simulink model "minJerk"  (R2014b)
settings: Solver=FixedStepDiscrete  StartTime=0.0  StopTime=100  FixedStep=0.01  RelTol=1e-3
InitFcn:
  | Plant_IC=0.0;
  | Plant_Min=-100.0;
  | Plant_Max=100.0;
  | Compensator_Kp=10.0;
  | Compensator_Ki=1.0;
  | AutoCompensator_ThresHystMax=0.05;
  | AutoCompensator_ThresHystMin=0.005;
  | ErrorStatisticsTimeWindow=1.0;
undefined symbols (not defined in the file or in its folder): CompensatorState
libraries: simulink x1, powerlib_meascontrol x1, dspbuff3 x1, dspstat3 x1, discretizing x1
settings Model: Creator=Ugo Pattacini  LastModifiedBy=Ugo Pattacini
settings OptimizationCC: OptimizeModelRefInitCode=on  LifeSpan=1
settings RTWCC: SystemTargetFile=ert.tlc  GenCodeOnly=on  TemplateMakefile=ert_default_tmf  Description=Embedded Coder  GenerateReport=on  ProcessScript=ert_make_rtw_hook  BuildConfiguration=Faster Runs  IncludeHyperlinkInReport=on  LaunchReport=on  TargetLang=C++
settings CodeAppCC: IgnoreCustomStorageClasses=off
settings ERTTargetCC: TargetLangStandard=C++03 (ISO)  GenerateSampleERTMain=on  MultiInstanceERTCode=on  CodeInterfacePackaging=Reusable function  ERTCustomFileTemplate=example_file_process.tlc

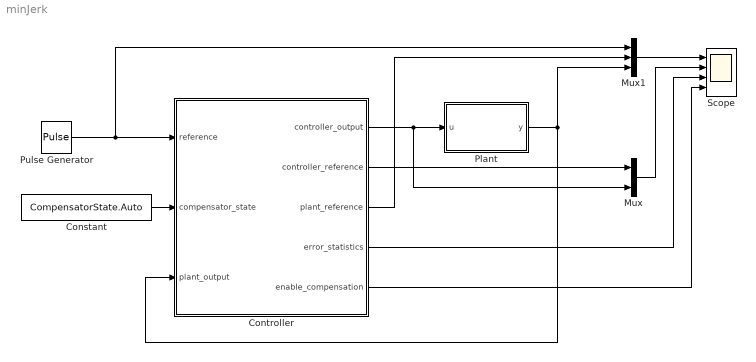
== system minJerk ==
  Constant : Constant  Value=CompensatorState.Auto  OutDataTypeStr=Enum: CompensatorState
  Controller : Subsystem
  Mux : Mux  Inputs=2
  Mux1 : Mux  Inputs=3
  Plant : Subsystem  TreatAsAtomicUnit=on  RTWFcnName=Plant
      settings: RTWFcnNameOpts=User specified
  Pulse Generator : DiscretePulseGenerator  PulseType=Time based  Period=20  PulseWidth=50
  Scope : Scope  NumInputPorts=4
      settings: TimeRange=100  YMin=-0.5~-2~0~-1  YMax=1.5~2~0.15~2
  wires:
  Pulse Generator/1 -> Mux1/1, Controller/1(reference)
  Controller/2(controller_reference) -> Mux/1
  Controller/3(plant_reference) -> Mux1/2
  Mux1/1 -> Scope/1
  Controller/1(controller_output) -> Mux/2, Plant/1(u)
  Plant/1(y) -> Mux1/3, Controller/3(plant_output)
  Mux/1 -> Scope/2
  Constant/1 -> Controller/2(compensator_state)
  Controller/4(error_statistics) -> Scope/3
  Controller/5(enable_compensation) -> Scope/4

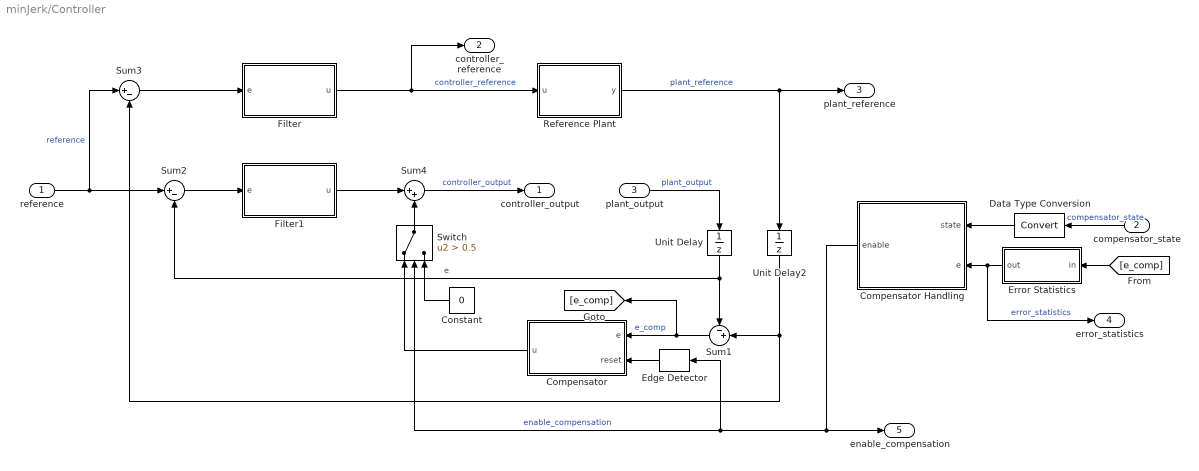
== system minJerk/Controller ==
  reference : Inport
  compensator_state : Inport  Port=2  OutDataTypeStr=Enum: CompensatorState
  plant_output : Inport  Port=3
  Compensator : Subsystem  TreatAsAtomicUnit=on  RTWFcnName=Compensator
      settings: RTWFcnNameOpts=User specified
  Compensator Handling : Stateflow chart  TreatAsAtomicUnit=on
  Constant : Constant  Value=0
  Data Type Conversion : DataTypeConversion
  Edge Detector : powerlib_meascontrol/Logic/Edge Detector  model=Rising  ic=0  Ts=-1
  Error Statistics : Subsystem  TreatAsAtomicUnit=on  RTWFcnName=ErrorStatistics
      settings: RTWFcnNameOpts=User specified
  Filter : Subsystem  TreatAsAtomicUnit=on  RTWFcnName=Filter
      settings: RTWFcnNameOpts=User specified
  Filter1 : Subsystem  TreatAsAtomicUnit=on  RTWFcnName=Filter
      settings: RTWFcnNameOpts=User specified
  Reference Plant : Subsystem  TreatAsAtomicUnit=on  RTWFcnName=ReferencePlant
      settings: RTWFcnNameOpts=User specified
  Sum1 : Sum  Inputs=-+|
  Sum2 : Sum  Inputs=|+-
  Sum3 : Sum  Inputs=|+-
  Sum4 : Sum  Inputs=|++
  Switch : Switch  Criteria=u2 > Threshold  Threshold=0.5
  Unit Delay : UnitDelay  InitialCondition=Plant_IC  SampleTime=-1
  Unit Delay2 : UnitDelay  InitialCondition=Plant_IC  SampleTime=-1
  controller_output : Outport
  controller_reference : Outport  Port=2
  plant_reference : Outport  Port=3
  error_statistics : Outport  Port=4
  enable_compensation : Outport  Port=5
  wires:
  Sum4/1 -> controller_output/1  "controller_output"
  reference/1 -> Sum2/1, Sum3/1  "reference"
  Filter1/1(u) -> Sum4/1
  Sum2/1 -> Filter1/1(e)
  Unit Delay/1 -> Sum2/2, Sum1/1  "e"
  Unit Delay2/1 -> Sum3/2, Sum1/2
  Reference Plant/1(y) -> plant_reference/1, Unit Delay2/1  "plant_reference"
  plant_output/1 -> Unit Delay/1  "plant_output"
  Compensator/1(u) -> Switch/1
  Filter/1(u) -> controller_reference/1, Reference Plant/1(u)  "controller_reference"
  Sum3/1 -> Filter/1(e)
  Sum1/1 -> [e_comp], Compensator/1(e)  "e_comp"
  Switch/1 -> Sum4/2
  Constant/1 -> Switch/3
  Compensator Handling/1(enable) -> Edge Detector/1, Switch/2, enable_compensation/1  "enable_compensation"
  Edge Detector/1 -> Compensator/2(reset)
  compensator_state/1 -> Data Type Conversion/1  "compensator_state"
  Error Statistics/1(out) -> error_statistics/1, Compensator Handling/2(e)  "error_statistics"
  [e_comp] -> Error Statistics/1(in)
  Data Type Conversion/1 -> Compensator Handling/1(state)

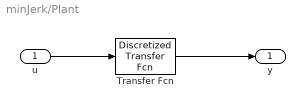
== system minJerk/Plant ==
  u : Inport
  Transfer Fcn : discretizing/Discretized Transfer Fcn  Numerator=[0.9]  Denominator=[0.5 1 0]  AbsTol=auto  SampleTime=0.01  method=tustin  Wc=0
  y : Outport
  wires:
  Transfer Fcn/1 -> y/1
  u/1 -> Transfer Fcn/1

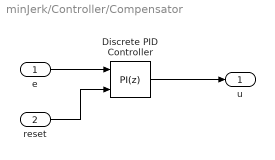
== system minJerk/Controller/Compensator ==
  e : Inport
  reset : Inport  Port=2
  Discrete PID Controller : simulink/Continuous/PID Controller  Controller=PI  TimeDomain=Discrete-time  SampleTime=0.01  IntegratorMethod=Trapezoidal  FilterMethod=Forward Euler  Form=Parallel  P=Compensator_Kp  I=Compensator_Ki  D=0  N=100  InitialConditionSource=internal  InitialConditionForIntegrator=0  InitialConditionForFilter=0  ExternalReset=rising  LimitOutput=off  UpperSaturationLimit=Plant_Max  LowerSaturationLimit=Plant_Min  LinearizeAsGain=off  AntiWindupMode=back-calculation  Kb=2  TrackingMode=off  Kt=1  PParamMin=[]  PParamMax=[]  IParamMin=[]  IParamMax=[]  DParamMin=[]  DParamMax=[]  NParamMin=[]  NParamMax=[]  KbParamMin=[]  KbParamMax=[]  KtParamMin=[]  KtParamMax=[]  POutMin=[]  POutMax=[]  IOutMin=[]  IOutMax=[]  DOutMin=[]  DOutMax=[]  NOutMin=[]  NOutMax=[]  KbOutMin=[]  KbOutMax=[]  KtOutMin=[]  KtOutMax=[]  IntegratorOutMin=[]  IntegratorOutMax=[]  FilterOutMin=[]  FilterOutMax=[]  SumOutMin=[]  SumOutMax=[]  SumI1OutMin=[]  SumI1OutMax=[]  SumI2OutMin=[]  SumI2OutMax=[]  SumI3OutMin=[]  SumI3OutMax=[]  SumDOutMin=[]  SumDOutMax=[]  SaturationOutMin=[]  SaturationOutMax=[]  IntegratorContinuousStateAttributes=''  IntegratorStateMustResolveToSignalObject=off  IntegratorRTWStateStorageClass=Auto  FilterContinuousStateAttributes=''  FilterStateMustResolveToSignalObject=off  FilterRTWStateStorageClass=Auto  DifferentiatorICPrevScaledInput=0  DifferentiatorOutMin=[]  DifferentiatorOutMax=[]  UseFilter=on
  u : Outport
  wires:
  e/1 -> Discrete PID Controller/1
  Discrete PID Controller/1 -> u/1
  reset/1 -> Discrete PID Controller/2

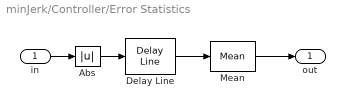
== system minJerk/Controller/Error Statistics ==
  in : Inport
  Abs : Abs
  Delay Line : dspbuff3/Delay Line  siz=ceil(ErrorStatisticsTimeWindow/0.01)  ic=0  directfeed=off  enable_output=off  hold_output=off  TreatMby1Signals=One channel
  Mean : dspstat3/Mean  run=off  reset_popup=None  InputProcessing=Columns as channels (frame based)  directionMode=Entire input  dimension=1  treatSBRowAsCol=on  roiEnable=off  roiType=Rectangles  roiPortion=Entire ROI  roiOutput=Individual statistics for each ROI  roiFlag=off  outputDataTypeStr=Inherit: Same as accumulator  outputLastDataTypeStr=Inherit: Same as accumulator  outputMin=[]  outputMax=[]  roundingMode=Floor  overflowMode=off
  out : Outport
  wires:
  in/1 -> Abs/1
  Delay Line/1 -> Mean/1
  Abs/1 -> Delay Line/1
  Mean/1 -> out/1

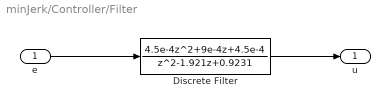
== system minJerk/Controller/Filter ==
  e : Inport
  Discrete Filter : DiscreteTransferFcn  Numerator=[4.5e-4 9e-4 4.5e-4]  Denominator=[1 -1.921 0.9231]  SampleTime=0.01
  u : Outport
  wires:
  Discrete Filter/1 -> u/1
  e/1 -> Discrete Filter/1

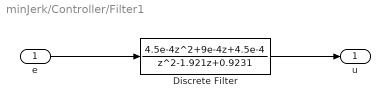
== system minJerk/Controller/Filter1 ==
  e : Inport
  Discrete Filter : DiscreteTransferFcn  Numerator=[4.5e-4 9e-4 4.5e-4]  Denominator=[1 -1.921 0.9231]  SampleTime=0.01
  u : Outport
  wires:
  e/1 -> Discrete Filter/1
  Discrete Filter/1 -> u/1

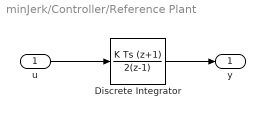
== system minJerk/Controller/Reference Plant ==
  u : Inport
  Discrete Integrator : DiscreteIntegrator  IntegratorMethod=Integration: Trapezoidal  InitialCondition=Plant_IC  InitialConditionSetting=State (most efficient)  SampleTime=0.01  LimitOutput=on  UpperSaturationLimit=Plant_Max  LowerSaturationLimit=Plant_Min
  y : Outport
  wires:
  Discrete Integrator/1 -> y/1
  u/1 -> Discrete Integrator/1

== stateflow chart minJerk/Controller/Compensator Handling ==
  state Select
  state AutomaticOff
    entry:
    enable=false;
  state AutomaticOn
    entry:
    enable=true;
  AutomaticOn -> Select [order 1] : [state!=Auto]
  (default) -> Select
  AutomaticOff -> Select [order 1] : [state!=Auto]
  (junction 13) -> Select [order 1] : [state==Off]
      | { enable=false; }
  (junction 13) -> Select [order 2] : [state==On]
      | { enable=true; }
  Select -> (junction 13)
  (junction 13) -> (junction 25) [order 3]
  (junction 25) -> AutomaticOff [order 2]
  (junction 25) -> AutomaticOn [order 1] : [e>AutoCompensator_ThresHystMax]
  AutomaticOff -> AutomaticOn [order 2] : [e>AutoCompensator_ThresHystMax]
  AutomaticOn -> AutomaticOff [order 2] : [e<AutoCompensator_ThresHystMin]
  data: state input Enum: CompensatorState; enable output boolean; e input; AutoCompensator_ThresHystMax parameter double; AutoCompensator_ThresHystMin parameter double
